simulink model "motor"  (R2013a)
settings: Solver=ode5  StartTime=0.0  StopTime=inf  RelTol=1e-3
values from neighbouring files (symbols this model uses):
  id_motor =     [LAB02_IDENT.mat]    (also in LAB02_IDENT_02.mat; data_ideal_motor_1.mat)
undefined symbols (not defined in the file or in its folder): National_Instruments, PCI
libraries: rtwinlib x2, dsparch4 x1
settings Model: SimulationMode=external  Creator=u_labelectro  LastModifiedBy=u_labelectro
settings HardwareCC: ProdIntDivRoundTo=Zero  ProdEndianess=LittleEndian  ProdHWDeviceType=Generic->32-bit x86 compatible
settings RTWCC: SystemTargetFile=rtwin.tlc  TemplateMakefile=rtwin.tmf  Description=Real-Time Windows Target  ProcessScript=rtwin_make_rtw_hook  RTWCompilerOptimization=On
settings CodeAppCC: MaxIdLength=95
settings RTWinTargetCC: TargetLibSuffix=_rtwin.lib  TargetPreCompLibLocation=D:\Real Time\toolbox\rtw\targets\rtwin\lib\win64  CodeReplacementLibrary=ANSI_C  RTWinDir=D:/REALTI~1/toolbox/rtw/targets/rtwin  TargetArch=win64

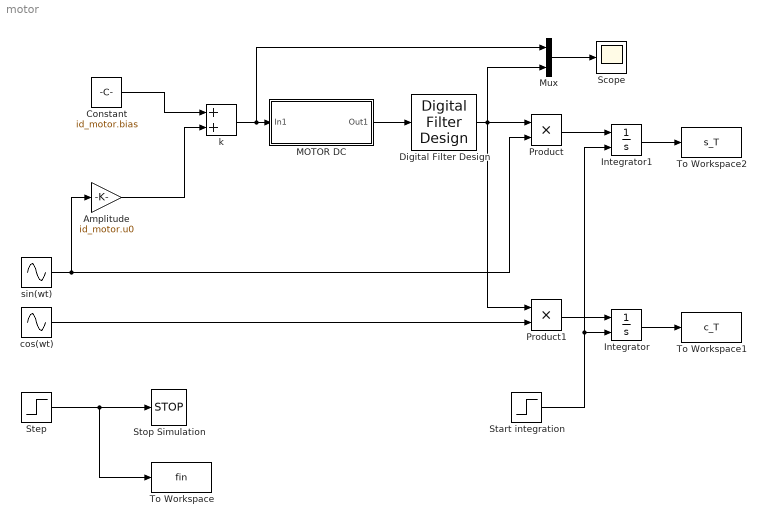
== system motor ==
  Amplitude : Gain  Gain=id_motor.u0
  Constant : Constant  Value=id_motor.bias
  Digital Filter Design : dsparch4/Digital Filter Design  mwdsp_browser_bugfix_var=off
  Integrator : Integrator  ExternalReset=rising
  Integrator1 : Integrator  ExternalReset=rising
  "MOTOR DC " : Subsystem  TreatAsAtomicUnit=on
  Mux : Mux  Inputs=2
  Product : Product
  Product1 : Product
  Scope : Scope
      settings: TimeRange=10  YMin=-10  YMax=10
  Start integration : Step  Time=id_motor.Tstart  SampleTime=0
  Step : Step  Time=id_motor.Tstop  SampleTime=0
  Stop Simulation : Stop
  To Workspace : ToWorkspace  VariableName=fin  SampleTime=-1  SaveFormat=Timeseries
  To Workspace1 : ToWorkspace  VariableName=c_T  SampleTime=-1
  To Workspace2 : ToWorkspace  VariableName=s_T  SampleTime=-1
  cos(wt) : Sin  Frequency=id_motor.w  Phase=pi/2  Samples=id_motor.w/id_motor.s  SampleTime=id_motor.s  Offset=5
  k : Sum
  sin(wt) : Sin  Frequency=id_motor.w  Samples=(id_motor.w)/(id_motor.s)  SampleTime=id_motor.s
  wires:
  Step/1 -> To Workspace/1, Stop Simulation/1
  Constant/1 -> k/1
  Amplitude/1 -> k/2
  Digital Filter Design/1 -> Mux/2, Product/1, Product1/1
  "MOTOR DC "/1(Out1) -> Digital Filter Design/1
  k/1 -> Mux/1, "MOTOR DC "/1(In1)
  Product/1 -> Integrator1/1
  Product1/1 -> Integrator/1
  Start integration/1 -> Integrator/2, Integrator1/2
  sin(wt)/1 -> Amplitude/1, Product/2
  cos(wt)/1 -> Product1/2
  Integrator1/1 -> To Workspace2/1
  Integrator/1 -> To Workspace1/1
  Mux/1 -> Scope/1

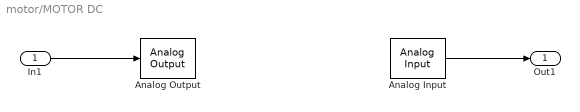
== system motor/MOTOR DC  ==
  In1 : Inport
  Analog Input : rtwinlib/Analog Input  SampleTime=0.01  MaxMissedTicks=10  ShowMissedTicks=off  YieldWhenWaiting=off  DrvName=National_Instruments/PCI-6229  DrvAddress=4294967295  DrvOptions=[0 0 0 0 0]  Channels=2  RangeMode=1  VoltRange=1  DataType=1
      settings: AttributesFormatString=National Instruments\nPCI-6229 [auto]
  Analog Output : rtwinlib/Analog Output  SampleTime=0.01  MaxMissedTicks=10  ShowMissedTicks=off  YieldWhenWaiting=off  DrvName=National_Instruments/PCI-6229  DrvAddress=4294967295  DrvOptions=[0 0 0 0 0]  Channels=1  RangeMode=1  VoltRange=1  InitialValue=[]  FinalValue=[]
      settings: AttributesFormatString=National Instruments\nPCI-6229 [auto]
  Out1 : Outport
  wires:
  Analog Input/1 -> Out1/1
  In1/1 -> Analog Output/1
